simulink model "keyborad_grabber"  (R2021a)
settings: Solver=VariableStepAuto  StartTime=0.0  StopTime=10.0  RelTol=1e-3
libraries: simulink x2, parrotlib x2
settings Model: Creator=s2130866  LastModifiedBy=s2130866

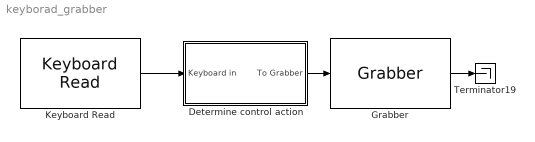
== system keyborad_grabber ==
  Determine control action : Subsystem
  Grabber : parrotlib/Grabber
      settings: SourceProductBaseCode=MINIDRONES
  Keyboard Read : parrotlib/Keyboard Read  SampleTime_=0.005
      settings: SourceProductBaseCode=MINIDRONES
  Terminator19 : Terminator
  wires:
  Determine control action/1(To Grabber) -> Grabber/1
  Grabber/1 -> Terminator19/1
  Keyboard Read/1 -> Determine control action/1("Keyboard in ")

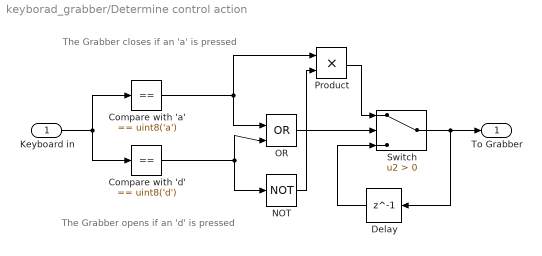
== system keyborad_grabber/Determine control action ==
  note: The Grabber closes if an 'a' is pressed
  note: The Grabber opens if an 'd' is pressed
  "Keyboard in " : Inport
  Compare with 'a' : simulink/Logic and Bit Operations/Compare To Constant  relop===  const=uint8('a')  OutDataTypeStr=boolean
  Compare with 'd' : simulink/Logic and Bit Operations/Compare To Constant  relop===  const=uint8('d')  OutDataTypeStr=boolean
  Delay : Delay  DelayLength=1
  NOT : Logic  Operator=NOT  IconShape=distinctive  AllPortsSameDT=off  OutDataTypeStr=boolean
  OR : Logic  Operator=OR  IconShape=distinctive  AllPortsSameDT=off  OutDataTypeStr=boolean
  Product : Product
  Switch : Switch  Criteria=u2 > Threshold
  To Grabber : Outport  VectorParamsAs1DForOutWhenUnconnected=off
  wires:
  Delay/1 -> Switch/3
  Compare with 'a'/1 -> OR/1, Product/1
  OR/1 -> Switch/2
  NOT/1 -> Product/2
  Switch/1 -> Delay/1, To Grabber/1
  "Keyboard in "/1 -> Compare with 'a'/1, Compare with 'd'/1
  Compare with 'd'/1 -> NOT/1, OR/2
  Product/1 -> Switch/1
